simulink model "VOO_First_Model"  (R2024a)
settings: Solver=FixedStepAuto  StartTime=0.0  StopTime=10  FixedStep=1e-3  RelTol=1e-3  EnableMultiTasking=on
undefined symbols (not defined in the file): D10, D11, D12, D2, D4, D5, D7, D8, D9, PTA0, PTA2, PTB23, PTB9, PTC3, PTC4, PTD0, PTD2, PTD3
libraries: frdmk64flib x9
settings Model: ExtModeTrigDuration=5  Creator=ryanb  LastModifiedBy=ryanb
settings OptimizationCC: EnhancedBackFolding=on  PassReuseOutputArgsAs=Individual arguments  ZeroExternalMemoryAtStartup=off  ZeroInternalMemoryAtStartup=off  MaxStackSize=64  OptimizeBlockOrder=speed  DifferentSizesBufferReuse=on  OptimizationCustomize=off  EfficientTunableParamExpr=on
settings DebuggingCC: ParameterTunabilityLossMsg=error
settings HardwareCC: ProdBitPerPointer=32  ProdBitPerSizeT=32  ProdBitPerPtrDiffT=32  ProdLargestAtomicInteger=Long  ProdLargestAtomicFloat=Double  ProdWordSize=32  ProdHWDeviceType=ARM Compatible->ARM Cortex
settings SFSimCC: MATLABDynamicMemAlloc=off
settings RTWCC: Description=Embedded Coder  SystemTargetFile=ert.tlc  HardwareBoard=NXP FRDM-K64F  TLCOptions="-aInlineSetEventsForThisBaseRateFcn=TLC_FALSE -aSuppressMultiTaskScheduler=TLC_FALSE  -aRateBasedStepFcn=0"  TemplateMakefile=ert_default_tmf  Toolchain=GNU Tools for ARM Embedded Processors
settings CodeAppCC: ForceParamTrailComments=on  IgnoreCustomStorageClasses=off  OperatorAnnotations=on  SimulinkDataObjDesc=on  SFDataObjDesc=on  InsertBlockDesc=on
settings ERTTargetCC: ExtModeTransport=4  ExtModeMexFile=sendToCommService

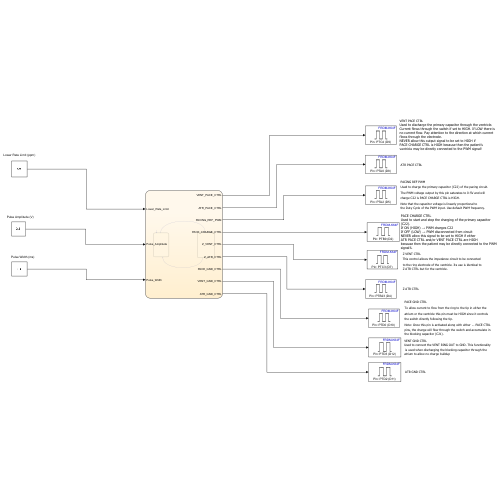
[thumbnail: Simulink's stored preview of the top-level diagram]
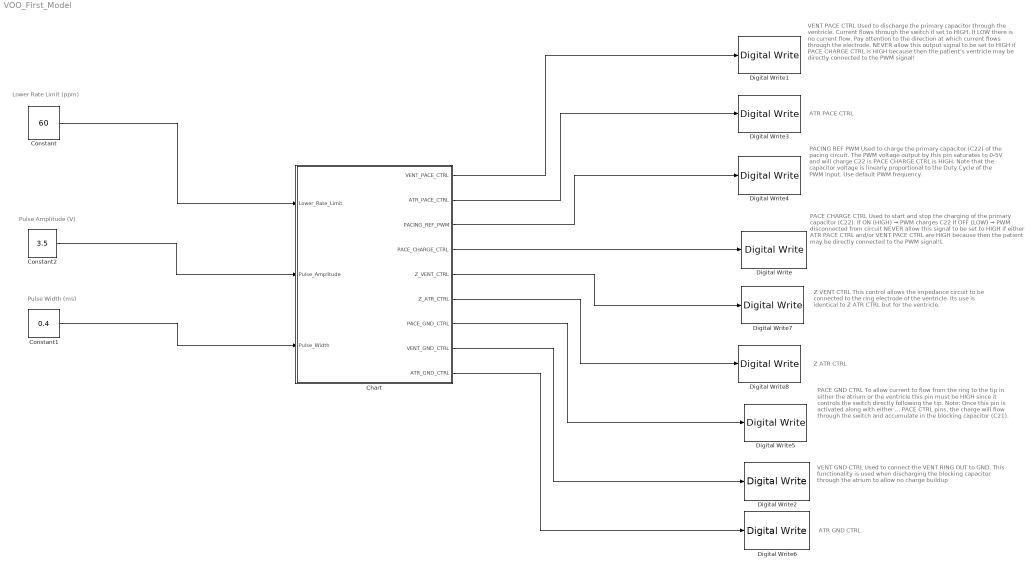
== system VOO_First_Model ==
  note: Pulse Amplitude (V)
  note: Pulse Width (ms)
  note: Lower Rate Limit (ppm)
  note: Z VENT CTRL
      | This control allows the impedance circuit to be connected
      | to the ring electrode of the ventricle. Its use is identical to
      | Z ATR CTRL but for the ventricle.
  note: PACE GND CTRL
      | To allow current to flow from the ring to the tip in either the
      | atrium or the ventricle this pin must be HIGH since it controls
      | the switch directly following the tip.
      | Note: Once this pin is activated along with either ... PACE CTRL
      | pins, the charge will flow through the switch and accumulate in
      | the blocking capacitor (C21).
  note: PACING REF PWM
      | Used to charge the primary capacitor (C22) of the pacing circuit.
      | The PWM voltage output by this pin saturates to 0-5V and will
      | charge C22 is PACE CHARGE CTRL is HIGH.
      | Note that the capacitor voltage is linearly proportional to
      | the Duty Cycle of the PWM input. Use default PWM frequency.
  note: VENT GND CTRL
      | Used to connect the VENT RING OUT to GND. This functionality
      | is used when discharging the blocking capacitor through the
      | atrium to allow no charge buildup
  note: VENT PACE CTRL
      | Used to discharge the primary capacitor through the ventricle.
      | Current flows through the switch if set to HIGH. If LOW there is
      | no current flow. Pay attention to the direction at which current
      | flows through the electrode.
      | NEVER allow this output signal to be set to HIGH if
      | PACE CHARGE CTRL is HIGH because then the patient’s
      | ventricle may be directly connected to the PWM signal!
  note: PACE CHARGE CTRL
      | Used to start and stop the charging of the primary capacitor
      | (C22).
      | If ON (HIGH) → PWM charges C22
      | If OFF (LOW) → PWM disconnected from circuit
      | NEVER allow this signal to be set to HIGH if either
      | ATR PACE CTRL and/or VENT PACE CTRL are HIGH
      | because then the patient may be directly connected to the PWM
      | signal!L
  note: ATR PACE CTRL
  note: ATR GND CTRL
  note: Z ATR CTRL
  Chart : Stateflow chart  TreatAsAtomicUnit=on
  Constant : Constant  Value=60
  Constant1 : Constant  Value=0.4
  Constant2 : Constant  Value=3.5
  Digital Write : frdmk64flib/Digital Write  Whichpin=PTB9 (D2)
  Digital Write1 : frdmk64flib/Digital Write  Whichpin=PTC4 (D9)
  Digital Write2 : frdmk64flib/Digital Write  Whichpin=PTD3 (D12)
  Digital Write3 : frdmk64flib/Digital Write  Whichpin=PTA0 (D8)
  Digital Write4 : frdmk64flib/Digital Write  Whichpin=PTA2 (D5)
  Digital Write5 : frdmk64flib/Digital Write  Whichpin=PTD0 (D10)
  Digital Write6 : frdmk64flib/Digital Write  Whichpin=PTD2 (D11)
  Digital Write7 : frdmk64flib/Digital Write  Whichpin=PTC3 (D7)
  Digital Write8 : frdmk64flib/Digital Write  Whichpin=PTB23 (D4)
  wires:
  Chart/1(VENT_PACE_CTRL) -> Digital Write1/1
  Chart/2(ATR_PACE_CTRL) -> Digital Write3/1
  Chart/3(PACING_REF_PWM) -> Digital Write4/1
  Chart/4(PACE_CHARGE_CTRL) -> Digital Write/1
  Chart/5(Z_VENT_CTRL) -> Digital Write7/1
  Chart/6(Z_ATR_CTRL) -> Digital Write8/1
  Chart/7(PACE_GND_CTRL) -> Digital Write5/1
  Chart/8(VENT_GND_CTRL) -> Digital Write2/1
  Chart/9(ATR_GND_CTRL) -> Digital Write6/1
  Constant/1 -> Chart/1(Lower_Rate_Limit)
  Constant1/1 -> Chart/3(Pulse_Width)
  Constant2/1 -> Chart/2(Pulse_Amplitude)

== stateflow chart VOO_First_Model/Chart ==
  state PACING
    entry:
    PACE_CHARGE_CTRL = 0;
    PACE_GND_CTRL = 1;
    ATR_PACE_CTRL = 0;
    ATR_GND_CTRL = 0;
    Z_ATR_CTRL = 0;
    Z_VENT_CTRL = 0;
    VENT_GND_CTRL = 0;
    VENT_PACE_CTRL = 1;
  state CHARGING
    entry:
    %%Charging C22
    ATR_PACE_CTRL = 0;
    VENT_PACE_CTRL = 0;
    PACE_CHARGE_CTRL = 1;
    %%Discharging Blocking Cap
    PACE_GND_CTRL = 1;
    Z_ATR_CTRL = 0;
    Z_VENT_CTRL = 0;
    ATR_GND_CTRL = 0;
    VENT_GND_CTRL = 1;
    PACING_REF_PWM = (Pulse_Amplitude/5.0)*100;
  CHARGING -> PACING : %%Pace Ready
      | [after(1/(Lower_Rate_Limit/60) - Pulse_Width/1000, sec)]
  (default) -> CHARGING
  PACING -> CHARGING : %%Recharge Ready
      | [after(Pulse_Width/1000, sec)]
  data: VENT_PACE_CTRL output; ATR_PACE_CTRL output; PACING_REF_PWM output; PACE_CHARGE_CTRL output; Z_VENT_CTRL output; Z_ATR_CTRL output; PACE_GND_CTRL output; VENT_GND_CTRL output; ATR_GND_CTRL output; Lower_Rate_Limit input; Pulse_Amplitude input; Pulse_Width input
